simulink model "robot_model"  (R2022a)
settings: Solver=VariableStepAuto  StartTime=0.0  StopTime=10.0  RelTol=1e-3
values from neighbouring files (symbols this model uses):
  b_actual_ft = 1    [run_robot_model.m]    (also in run_steeringsimulation.m; run_steeringsimulation_simple.m)
  counts_to_rad = 1/rad_to_counts    (= 0.00174532925199)    [run_robot_model.m]    (also in run_steeringsimulation.m; run_steeringsimulation_simple.m)
  K_l = 1    [run_robot_model.m]    (also in run_steeringsimulation.m = 1.1; run_steeringsimulation_simple.m)
  K_r = 1.5    [run_robot_model.m]    (also in run_steeringsimulation.m = 1; run_steeringsimulation_simple.m = 1)
  r_actual_ft = .5    (= 0.5)    [run_robot_model.m]    (also in run_steeringsimulation.m; run_steeringsimulation_simple.m)
  rad_to_counts = 3600/(2*pi)    (= 572.957795131)    [run_robot_model.m]    (also in run_steeringsimulation.m; run_steeringsimulation_simple.m)
  sigma_l = 10    [run_robot_model.m]    (also in run_steeringsimulation.m = 13; run_steeringsimulation_simple.m)
  sigma_r = 15    [run_robot_model.m]    (also in run_steeringsimulation.m = 10; run_steeringsimulation_simple.m = 10)
  Ts = .01    (= 0.01)    [run_robot_model.m]    (also in run_steeringsimulation.m; run_steeringsimulation_simple.m)
libraries: simulink x2
settings Model: Creator=tvincent  LastModifiedBy=tvincent

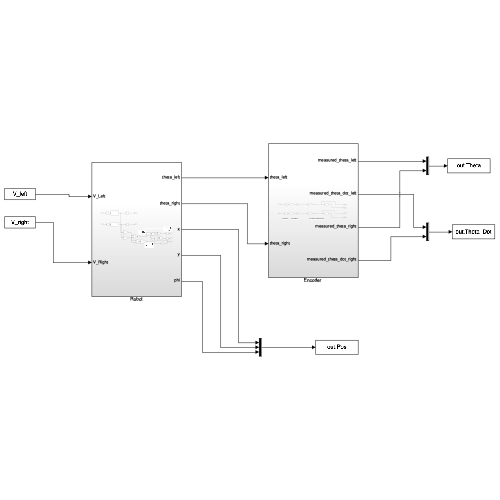
[thumbnail: Simulink's stored preview of the top-level diagram]
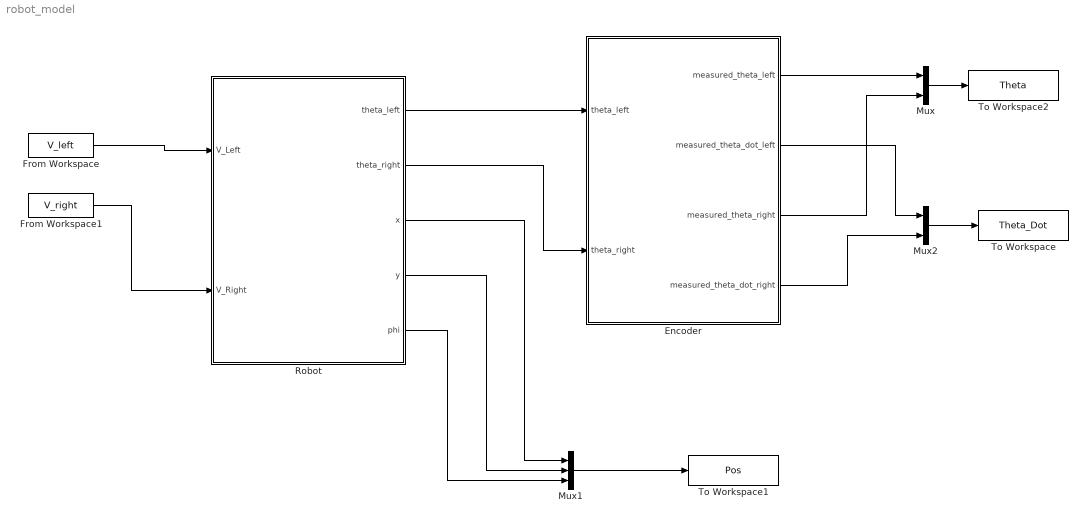
== system robot_model ==
  "Encoder " : Subsystem
  From Workspace : FromWorkspace  VariableName=V_left
  From Workspace1 : FromWorkspace  VariableName=V_right
  Mux : Mux  Inputs=2
  Mux1 : Mux  Inputs=3
  Mux2 : Mux  Inputs=2
  Robot : Subsystem
  To Workspace : ToWorkspace  VariableName=Theta_Dot  SaveFormat=Timeseries  SampleTime=.01
  To Workspace1 : ToWorkspace  VariableName=Pos  SaveFormat=Timeseries  SampleTime=.1
  To Workspace2 : ToWorkspace  VariableName=Theta  SaveFormat=Timeseries  SampleTime=.01
  wires:
  From Workspace/1 -> Robot/1(V_Left)
  From Workspace1/1 -> Robot/2(V_Right)
  Mux1/1 -> To Workspace1/1
  Robot/3(x) -> Mux1/1
  Robot/4(y) -> Mux1/2
  Robot/5(phi) -> Mux1/3
  Robot/1(theta_left) -> "Encoder "/1(theta_left)
  Robot/2(theta_right) -> "Encoder "/2(theta_right)
  "Encoder "/1(measured_theta_left) -> Mux/1
  "Encoder "/4(measured_theta_dot_right) -> Mux2/2
  "Encoder "/3(measured_theta_right) -> Mux/2
  "Encoder "/2(measured_theta_dot_left) -> Mux2/1
  Mux/1 -> To Workspace2/1
  Mux2/1 -> To Workspace/1

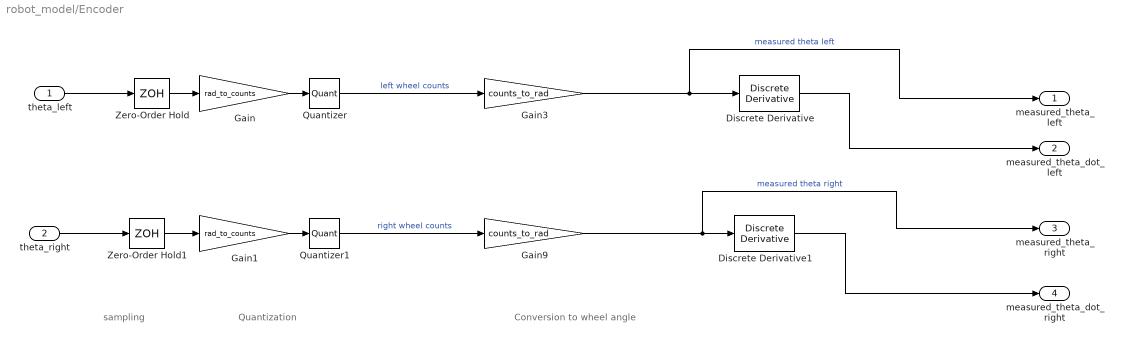
== system robot_model/Encoder  ==
  note: sampling
  note: Quantization
  note: Conversion to wheel angle
  theta_left : Inport
  theta_right : Inport  Port=2
  Discrete Derivative : simulink/Discrete/Discrete Derivative  gainval=1  ICPrevScaledInput=0.0  OutMin=[]  OutMax=[]  OutDataType=fixdt(1, 16)  OutScaling=2^-10  DoSatur=off
  Discrete Derivative1 : simulink/Discrete/Discrete Derivative  gainval=1  ICPrevScaledInput=0.0  OutMin=[]  OutMax=[]  OutDataType=fixdt(1, 16)  OutScaling=2^-10  DoSatur=off
  Gain : Gain  Gain=rad_to_counts
  Gain1 : Gain  Gain=rad_to_counts
  Gain3 : Gain  Gain=counts_to_rad
  Gain9 : Gain  Gain=counts_to_rad
  Quantizer : Quantizer  QuantizationInterval=1
  Quantizer1 : Quantizer  QuantizationInterval=1
  Zero-Order Hold : ZeroOrderHold  SampleTime=Ts
  Zero-Order Hold1 : ZeroOrderHold  SampleTime=Ts
  measured_theta_left : Outport
  measured_theta_dot_left : Outport  Port=2
  measured_theta_right : Outport  Port=3
  measured_theta_dot_right : Outport  Port=4
  wires:
  Zero-Order Hold/1 -> Gain/1
  Gain/1 -> Quantizer/1
  Quantizer/1 -> Gain3/1  "left wheel counts"
  Gain3/1 -> measured_theta_left/1, Discrete Derivative/1  "measured theta left"
  Quantizer1/1 -> Gain9/1  "right wheel counts"
  Zero-Order Hold1/1 -> Gain1/1
  Gain1/1 -> Quantizer1/1
  Gain9/1 -> measured_theta_right/1, Discrete Derivative1/1  "measured theta right"
  Discrete Derivative/1 -> measured_theta_dot_left/1
  Discrete Derivative1/1 -> measured_theta_dot_right/1
  theta_left/1 -> Zero-Order Hold/1
  theta_right/1 -> Zero-Order Hold1/1

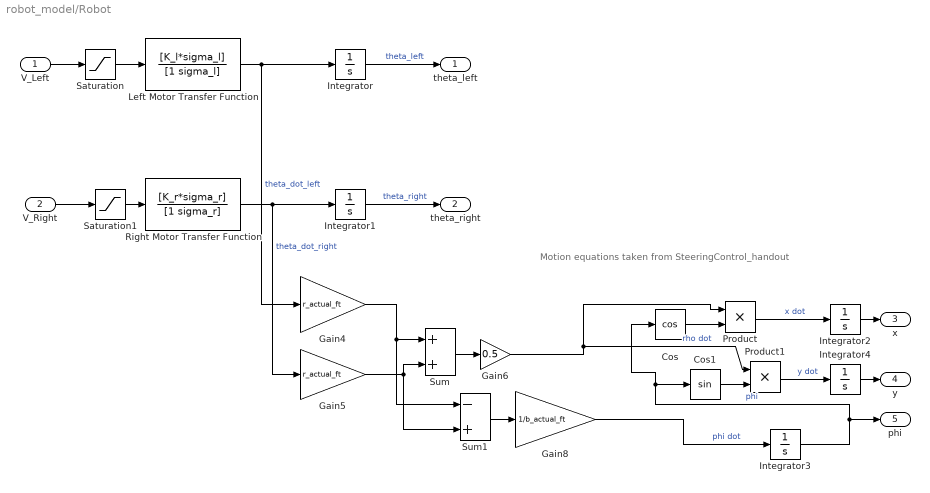
== system robot_model/Robot ==
  note: Motion equations taken from SteeringControl_handout
  V_Left : Inport
  V_Right : Inport  Port=2
  Cos : Trigonometry  Operator=cos
  Cos1 : Trigonometry
  Gain4 : Gain  Gain=r_actual_ft
  Gain5 : Gain  Gain=r_actual_ft
  Gain6 : Gain  Gain=0.5
  Gain8 : Gain  Gain=1/b_actual_ft
  Integrator{,1..4} (5 alike) : Integrator
  Left Motor Transfer Function : TransferFcn  Numerator=[K_l*sigma_l]  Denominator=[1 sigma_l]
  Product : Product
  Product1 : Product
  Right Motor Transfer Function : TransferFcn  Numerator=[K_r*sigma_r]  Denominator=[1 sigma_r]
  Saturation : Saturate  UpperLimit=7.5  LowerLimit=-7.5
  Saturation1 : Saturate  UpperLimit=7.5  LowerLimit=-7.5
  Sum : Sum
  Sum1 : Sum  Inputs=-+
  theta_left : Outport
  theta_right : Outport  Port=2
  x : Outport  Port=3
  y : Outport  Port=4
  phi : Outport  Port=5
  wires:
  V_Left/1 -> Saturation/1
  Left Motor Transfer Function/1 -> Gain4/1, Integrator/1  "theta_dot_left"
  Saturation/1 -> Left Motor Transfer Function/1
  V_Right/1 -> Saturation1/1
  Saturation1/1 -> Right Motor Transfer Function/1
  Right Motor Transfer Function/1 -> Gain5/1, Integrator1/1  "theta_dot_right"
  Sum/1 -> Gain6/1
  Integrator2/1 -> x/1
  Gain5/1 -> Sum/2, Sum1/2
  Sum1/1 -> Gain8/1
  Gain4/1 -> Sum1/1, Sum/1
  Integrator3/1 -> Cos1/1, Cos/1, phi/1  "phi"
  Gain8/1 -> Integrator3/1  "phi dot"
  Gain6/1 -> Product1/1, Product/1  "rho dot"
  Product/1 -> Integrator2/1  "x dot"
  Cos/1 -> Product/2
  Cos1/1 -> Product1/2
  Product1/1 -> Integrator4/1  "y dot"
  Integrator4/1 -> y/1
  Integrator/1 -> theta_left/1  "theta_left"
  Integrator1/1 -> theta_right/1  "theta_right"
